simulink model "Introduction_to_Simulink"  (R2015a)
settings: Solver=ode45  StartTime=0.0  StopTime=10.0  RelTol=1e-3
settings Model: Creator=pc  LastModifiedBy=pc

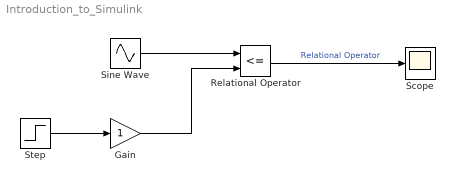
== system Introduction_to_Simulink ==
  Gain : Gain
  Relational Operator : RelationalOperator  Operator=<=  OutDataTypeStr=boolean
  Scope : Scope
  Sine Wave : Sin  SampleTime=0
  Step : Step  Time=2  SampleTime=0
  wires:
  Sine Wave/1 -> Relational Operator/1
  Gain/1 -> Relational Operator/2
  Step/1 -> Gain/1
  Relational Operator/1 -> Scope/1  "Relational Operator"
